simulink library "halout"  (R2021b)
settings: Solver=VariableStepAuto  StartTime=0.0  StopTime=10.0  RelTol=1e-3
undefined symbols (not defined in the file): C_TASK_5MS_S, FALSE, KHAL_CAN1TxReq_flg, KHAL_CAN2TxReq_flg, KHAL_CAN3FD3VCU1toNIDECTxReq_flg, KHAL_CAN3FD3VCU1TxReq_flg, KHAL_CAN3FD3VCU2E2E_flg, KHAL_CAN3FD3VCU2toNIDECE2E_flg, KHAL_CAN3FD3VCU2toNIDECTxReq_flg, KHAL_CAN3FD3VCU2TxReq_flg, KHAL_CAN3TxReq_flg, KHAL_CAN4FD4CE1000E2E_flg, KHAL_CAN4FD4CE1000TxReq_flg, KHAL_CAN4TxReq_flg, KHAL_CAN5TxReq_flg, KHAL_CAN7TxReq_flg, ONE_INT, TRUE, ZERO_INT
libraries: FVT_lib x258, simulink x115
(part 17 of 17)

== stateflow chart halout/HAL_OUT/CAN_Scheduler ==
  state CAN_scheduler
    (default) -> (junction 55)
    CAN_scheduler -> (junction 55)
    (junction 55) -> (junction 53) [order 1] : [KHAL_CAN1TxReq_flg && VOUTP_ALLCANTxReq_flg]
    (junction 55) -> (junction 214) [order 2]
    (junction 53) -> (junction 212) : {
        | trig_can1;
        | }
    (junction 212) -> (junction 214)
    (junction 214) -> (junction 250)
    (junction 250) -> (junction 251) [order 1] : [KHAL_CAN2TxReq_flg && VOUTP_ALLCANTxReq_flg]
    (junction 250) -> (junction 253) [order 2]
    (junction 251) -> (junction 247) : {
        | trig_can2;
        | }
    (junction 247) -> (junction 253)
    (junction 253) -> (junction 258)
    (junction 258) -> (junction 259) [order 1] : [KHAL_CAN3TxReq_flg && VOUTP_ALLCANTxReq_flg]
    (junction 258) -> (junction 261) [order 2]
    (junction 259) -> (junction 255) : {
        | trig_can3;
        | }
    (junction 255) -> (junction 261)
    (junction 261) -> (junction 266)
    (junction 266) -> (junction 267) [order 1] : [KHAL_CAN4TxReq_flg && VOUTP_ALLCANTxReq_flg]
    (junction 266) -> (junction 269) [order 2]
    (junction 267) -> (junction 263) : {
        | trig_can4;
        | }
    (junction 263) -> (junction 269)
    (junction 269) -> (junction 274)
    (junction 274) -> (junction 275) [order 1] : [KHAL_CAN5TxReq_flg && VOUTP_ALLCANTxReq_flg]
    (junction 274) -> (junction 277) [order 2]
    (junction 275) -> (junction 271) : {
        | trig_can5;
        | }
    (junction 271) -> (junction 277)
    (junction 277) -> (junction 323)
    (junction 323) -> (junction 322) [order 1] : [KHAL_CAN6TxReq_flg && VOUTP_ALLCANTxReq_flg]
    (junction 323) -> (junction 324) [order 2]
    (junction 322) -> (junction 321) : {
        | trig_can6;
        | }
    (junction 321) -> (junction 324)
  data: KHAL_CAN1TxReq_flg input; KHAL_CAN2TxReq_flg input; KHAL_CAN3TxReq_flg input; KHAL_CAN4TxReq_flg input; KHAL_CAN5TxReq_flg input; KHAL_CAN6TxReq_flg input; VOUTP_ALLCANTxReq_flg input
  events: trig_can1 output FUNCTION_CALL_EVENT; trig_can2 output FUNCTION_CALL_EVENT; trig_can3 output FUNCTION_CALL_EVENT; trig_can4 output FUNCTION_CALL_EVENT; trig_can5 output FUNCTION_CALL_EVENT; trig_can6 output FUNCTION_CALL_EVENT
